simulink model "PMDC_exhibition"  (R2023b)
settings: Solver=VariableStepAuto  StartTime=0.0  StopTime=140  RelTol=1e-3
undefined symbols (not defined in the file or in its folder): B, dt, dT, J, Ke, Kt, L, LoadMode, R, Ro, SlopeR, Ts, Vp, Vs
libraries: simulink x1
settings Model: Creator=yanqi  LastModifiedBy=Brian Cheng

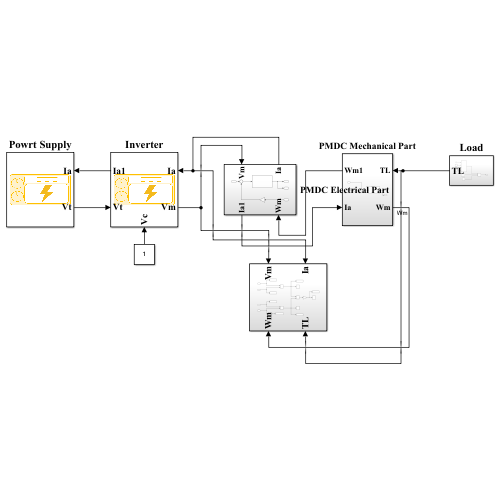
[thumbnail: Simulink's stored preview of the top-level diagram]
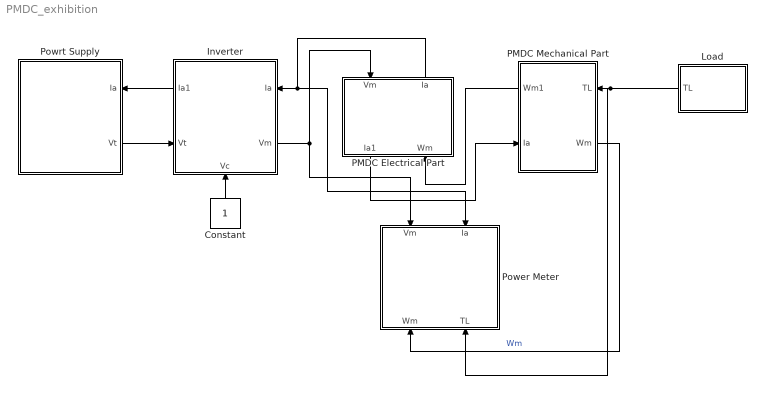
== system PMDC_exhibition ==
  Constant : Constant
  Inverter : Subsystem  InitFcn=Vp = 1;
      settings: PortSchema="{\"entries\":[{\"content\":{\"sides\":[{\"content\":{\"connectorIds\":[\"Out2\",\"In1\"]},\"type\":\"ConnectorPlacement.EquallySpacedRectSide\",\"uuid\":\"717e91a0-288b-4ba5-84da-f262c24688bc\"},{\"content\":{\"connectorIds\":[\"In3\",\"Out1\"],\"side\":\"RIGHT\"},\"type\":\"ConnectorPlacement.EquallySpacedRectSide\",\"uuid\":\"569ee505-38fb-400b-9e45-0fafedafb0f3\"},{\"content\":{\"side\":\"TOP\"},\"type\":\"ConnectorPlacement.EquallySpacedRectSide\",\"uuid\":\"44407c3d-239d-4fc9-b2d2-10ddbad2f525\"},{\"content\":{\"connectorIds\":[\"In2\"],\"side\":\"BOTTOM\"},\"type\":\"ConnectorPlacement.EquallySpacedRectSide\",\"uuid\":\"abc944a0-1837-407a-a5f0-1c34ab870232\"}]},\"type\":\"ConnectorPlacement.EquallySpacedConnector\",\"uuid\":\"e894aa65-7991-48d5-91da-50bab94327d3\"}],\"packageUris\":[\"http://schema.mathworks.com/mf0/Connector/R2020b\"],\"version\":\"1.0\"}"
      mask Display: image('$imagefile');
  Load : Subsystem  InitFcn=|
      | dt = 0.2;
      | dT = 0.05;
      | Ts = 2;
      | SlopeR = 0.2;
      | % if LoadMode>1.5, then use stair load
      | % if LoadMode<1.5, use linear load
      | LoadMode = 2;
  PMDC Electrical Part : Subsystem  InitFcn=|
      | % a=100
      | L = 0.0003137*a
      | R = 0.157378*a
      | J = 0.000466*a
      | B = 0.0002546*a
      | Ke = 0.0492*a
      | Kt = 0.0501*a
      settings: PortSchema="{\"entries\":[{\"content\":{\"sides\":[{\"content\":{\"connectorIds\":[\"Out2\",\"In1\"]},\"type\":\"ConnectorPlacement.EquallySpacedRectSide\",\"uuid\":\"0a5f02b8-770b-4e6c-8352-f728989d031b\"},{\"content\":{\"connectorIds\":[\"In2\",\"Out1\"],\"side\":\"RIGHT\"},\"type\":\"ConnectorPlacement.EquallySpacedRectSide\",\"uuid\":\"644f1108-5054-471c-8ace-4ff400685a6d\"},{\"content\":{\"connectorIds\":[],\"side\":\"TOP\"},\"type\":\"ConnectorPlacement.EquallySpacedRectSide\",\"uuid\":\"91f6ac77-69b1-43a4-9d17-8984b5c833f8\"}]},\"type\":\"ConnectorPlacement.EquallySpacedConnector\",\"uuid\":\"c8686663-a1fa-49f9-b914-1752eb8f4683\"}],\"packageUris\":[\"http://schema.mathworks.com/mf0/Connector/R2020b\"],\"version\":\"1.0\"}"
  PMDC Mechanical Part : Subsystem
      settings: PortSchema="{\"entries\":[{\"content\":{\"sides\":[{\"content\":{\"connectorIds\":[\"Out2\",\"In1\"]},\"type\":\"ConnectorPlacement.EquallySpacedRectSide\",\"uuid\":\"0a5f02b8-770b-4e6c-8352-f728989d031b\"},{\"content\":{\"connectorIds\":[\"In2\",\"Out1\"],\"side\":\"RIGHT\"},\"type\":\"ConnectorPlacement.EquallySpacedRectSide\",\"uuid\":\"644f1108-5054-471c-8ace-4ff400685a6d\"},{\"content\":{\"connectorIds\":[],\"side\":\"TOP\"},\"type\":\"ConnectorPlacement.EquallySpacedRectSide\",\"uuid\":\"91f6ac77-69b1-43a4-9d17-8984b5c833f8\"}]},\"type\":\"ConnectorPlacement.EquallySpacedConnector\",\"uuid\":\"c8686663-a1fa-49f9-b914-1752eb8f4683\"}],\"packageUris\":[\"http://schema.mathworks.com/mf0/Connector/R2020b\"],\"version\":\"1.0\"}"
  "Power Meter " : Subsystem  InitFcn=|  StopFcn=|
      InitFcn=|
      | %% ModePlot
      | % PlotMode=1 or 2
      | PlotMode = 2;
      StopFcn=|
      | % %% Data Loading
      | % 
      | % tl = out.Tl;
      | % f = size(tl);
      | % 
      | % % clear datas 
      | % torque = 0;
      | % y1 = 0; y2 = 0; y3 = 0; y4 = 0;
      | % 
      | % switch LoadMode   % mode ( 1:ramp load , 2:stair load )
      | % 
      | %     case 1  
      | % 
      | %         i = 1;
      | %         while 1
      | %             if tl(i) > 0.01
      | %                s = i;
      | %                break
      | %             end
      | %             i = i+1;
      | %         end
      | %         torque = out.Tl(s:f(1));
      | %         y1 = out.omega(s:f(1));
      | %         y2 = out.Eff(s:f(1));
      | %         y3 = out.Pin(s:f(1));
      | %         y4 = out.Pout(s:f(1));
      | %         case 2
      | % 
      | %         tl_pre = 0;
      | %         j = 1;
      | %         for i = 1:f(1)           
      | %             if tl(i) > tl_pre
      | %                 torque(j,1) = tl(i-1);
      | %                 y1(j,1) = out.omega((i-1),1);
      | %                 y2(j,1) = out.Eff((i-1),1);
      | %                 y3(j,1) = out.Pin((i-1),1);
      | %                 y4(j,1) = out.Pout((i-1),1);
      | %                 j = j+1;
      | %             end
      | %             tl_pre = tl(i);
      | %         end
      | % end
      | % 
      | % %% Plot
      | % % plot TN curve
      | % 
      | % figure(1);
      | % 
      | % % figure(2);
      | % clf;
      | % 
      | % % Create empty axis system with 4 y axis by calling:
      | % % handle = maxis(number of axis, y-spacing between outside lines)
      | % h = myaxisc(4,0.10,[0.1,0.1,0.8,0.8]); % Specify position
      | % 
      | % % Call plot and specify y-axis number using method h.p(nr). For creating a
      | % % legend later, we need to assign the handles returned by plot to p.
      | % switch PlotMode
      | % 
      | %     case 1  
      | %         p(1) = plot(h.p(1),torque,y1,'b','LineWidth',1.2);
      | %         p(2) = plot(h.p(2),torque,y2,'Color',[0.4660 0.6740 0.1880],'LineWidth',1.2);
      | %         p(3) = plot(h.p(3),torque,y3,'r','LineWidth',1.2);
      | %         p(4) = plot(h.p(4),torque,y4,'Color',[0.9290 0.6940 0.1250],'LineWidth',1.2);
      | %         print("case1");
      | % 
      | %     case 2
      | %         p(1) = plot(h.p(1),torque,y1,'b-*','LineWidth',1.1);
      | %         p(2) = plot(h.p(2),torque,y2,'-*','Color',[0.4660 0.6740 0.1880],'LineWidth',1.1);
      | %         p(3) = plot(h.p(3),torque,y3,'r-*','LineWidth',1.1);
      | %         p(4) = plot(h.p(4),torque,y4,'-*','Color',[0.9290 0.6940 0.1250],'LineWidth',1.1);
      | %         print("case2");
      | % 
      | % end
      | % 
      | % h.autoscale % Automatically Scale Y Axis
      | % 
      | % % Additional methods to modify appearance, scaling and so on:
      | % 
      | % h.autoy(3) % Autoscale only specified y-axis
      | % %h.ylim(3,[95,105]); % Set Y-Limits for axis 3
      | % l = size(torque);
      | % h.xlim([0,torque(l(1),1)+0.05]);
      | % h.ylim(2,[0,100]); % Set Y-Limits for axis 4
      | % 
      | % h.gridon % Enable grid (use h.gridoff to remove)
      | % 
      | % % Modify the y-Axis Color
      | % h.ycolor(1,'b');
      | % h.ycolor(2,[0.4660 0.6740 0.1880]);
      | % h.ycolor(3,'r');
      | % h.ycolor(4,[0.9290 0.6940 0.1250]);
      | % 
      | % % Add y-Labels
      | % h.ylabel(1,'Speed (RPM)');
      | % h.ylabel(2,'Efficiency (%)');
      | % h.ylabel(3,'Pin (W)');
      | % h.ylabel(4,'Pout (W)');
      | % 
      | % % Add x-Label
      | % h.xlabel('TL (Nm)');
      | % 
      | % % Change Position of the whole myaxisc-Object
      | % h.position([0.1,0.1,0.8,0.8],0.12); % Position-Vector and Spacing 0.12
      | % 
      | % % Change all font sizes
      | % h.fontsize(10)
      settings: PortSchema="{\"entries\":[{\"content\":{\"sides\":[{\"content\":{\"connectorIds\":[\"In1\",\"In2\"]},\"type\":\"ConnectorPlacement.EquallySpacedRectSide\",\"uuid\":\"e8c36156-32d4-4676-af0d-0891e0773ccb\"},{\"content\":{\"connectorIds\":[\"In3\",\"In4\"],\"side\":\"RIGHT\"},\"type\":\"ConnectorPlacement.EquallySpacedRectSide\",\"uuid\":\"5c876be3-b715-4990-b5f5-1fbda74411c9\"},{\"content\":{\"side\":\"TOP\"},\"type\":\"ConnectorPlacement.EquallySpacedRectSide\",\"uuid\":\"8aaa78a6-3767-49bf-860f-056d8a2101ef\"}]},\"type\":\"ConnectorPlacement.EquallySpacedConnector\",\"uuid\":\"6a38af7a-9eb4-49af-a88b-27cf70b05ead\"}],\"packageUris\":[\"http://schema.mathworks.com/mf0/Connector/R2020b\"],\"version\":\"1.0\"}"
  Powrt Supply : Subsystem  InitFcn=|
      | Vs = 110;
      | Ro = 0.001;
      settings: PortSchema="{\"entries\":[{\"content\":{\"sides\":[{\"content\":{},\"type\":\"ConnectorPlacement.EquallySpacedRectSide\",\"uuid\":\"717e91a0-288b-4ba5-84da-f262c24688bc\"},{\"content\":{\"connectorIds\":[\"In1\",\"Out1\"],\"side\":\"RIGHT\"},\"type\":\"ConnectorPlacement.EquallySpacedRectSide\",\"uuid\":\"569ee505-38fb-400b-9e45-0fafedafb0f3\"},{\"content\":{\"side\":\"TOP\"},\"type\":\"ConnectorPlacement.EquallySpacedRectSide\",\"uuid\":\"44407c3d-239d-4fc9-b2d2-10ddbad2f525\"}]},\"type\":\"ConnectorPlacement.EquallySpacedConnector\",\"uuid\":\"e894aa65-7991-48d5-91da-50bab94327d3\"}],\"packageUris\":[\"http://schema.mathworks.com/mf0/Connector/R2020b\"],\"version\":\"1.0\"}"
      mask Display: image('$imagefile');
  wires:
  Powrt Supply/1(Vt) -> Inverter/1(Vt)
  PMDC Electrical Part/2(Ia) -> "Power Meter "/1(Ia), Inverter/3(Ia)
  Inverter/1(Vm) -> "Power Meter "/2(Vm), PMDC Electrical Part/1(Vm)
  Load/1(TL) -> "Power Meter "/3(TL), PMDC Mechanical Part/2(TL)
  PMDC Mechanical Part/1(Wm) -> "Power Meter "/4(Wm)  "Wm"
  Constant/1 -> Inverter/2(Vc)
  Inverter/2(Ia1) -> Powrt Supply/1(Ia)
  PMDC Electrical Part/1(Ia1) -> PMDC Mechanical Part/1(Ia)
  PMDC Mechanical Part/2(Wm1) -> PMDC Electrical Part/2(Wm)

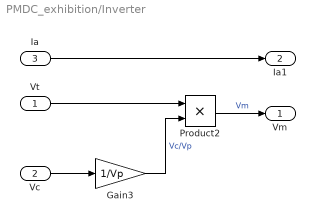
== system PMDC_exhibition/Inverter ==
  Vt : Inport
  Vc : Inport  Port=2
  Ia : Inport  Port=3
  Gain3 : Gain  Gain=1/Vp
  Product2 : Product
  Vm : Outport
  Ia1 : Outport  Port=2
  wires:
  Ia/1 -> Ia1/1
  Vc/1 -> Gain3/1
  Vt/1 -> Product2/1
  Product2/1 -> Vm/1  "Vm"
  Gain3/1 -> Product2/2  "Vc/Vp"

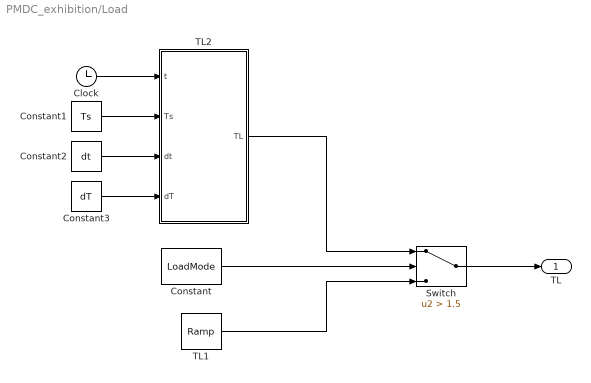
== system PMDC_exhibition/Load ==
  Clock : Clock
  Constant : Constant  Value=LoadMode
  Constant1 : Constant  Value=Ts
  Constant2 : Constant  Value=dt  SampleTime=dT
  Constant3 : Constant  Value=dT
  Switch : Switch  Criteria=u2 > Threshold  Threshold=1.5  SaturateOnIntegerOverflow=off  InputSameDT=off
  TL1 : simulink/Sources/Ramp  slope=SlopeR  start=Ts  InitialOutput=0
  TL2 : MATLAB Function  TreatAsAtomicUnit=on
  TL : Outport
  wires:
  Constant2/1 -> TL2/3(dt)
  Constant3/1 -> TL2/4(dT)
  Clock/1 -> TL2/1(t)
  Constant1/1 -> TL2/2(Ts)
  Switch/1 -> TL/1
  Constant/1 -> Switch/2
  TL2/1(TL) -> Switch/1
  TL1/1 -> Switch/3

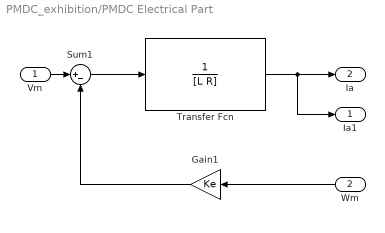
== system PMDC_exhibition/PMDC Electrical Part ==
  Vm : Inport
  Wm : Inport  Port=2
  Gain1 : Gain  Gain=Ke
  Sum1 : Sum  Inputs=|+-
  Transfer Fcn : TransferFcn  Denominator=[L R]
  Ia1 : Outport
  Ia : Outport  Port=2
  wires:
  Gain1/1 -> Sum1/2
  Sum1/1 -> Transfer Fcn/1
  Transfer Fcn/1 -> Ia1/1, Ia/1
  Wm/1 -> Gain1/1
  Vm/1 -> Sum1/1

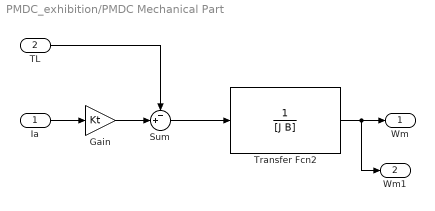
== system PMDC_exhibition/PMDC Mechanical Part ==
  Ia : Inport
  TL : Inport  Port=2
  Gain : Gain  Gain=Kt
  Sum : Sum  Inputs=-+|
  Transfer Fcn2 : TransferFcn  Denominator=[J B]
  Wm : Outport
  Wm1 : Outport  Port=2
  wires:
  Gain/1 -> Sum/2
  Ia/1 -> Gain/1
  Sum/1 -> Transfer Fcn2/1
  TL/1 -> Sum/1
  Transfer Fcn2/1 -> Wm1/1, Wm/1

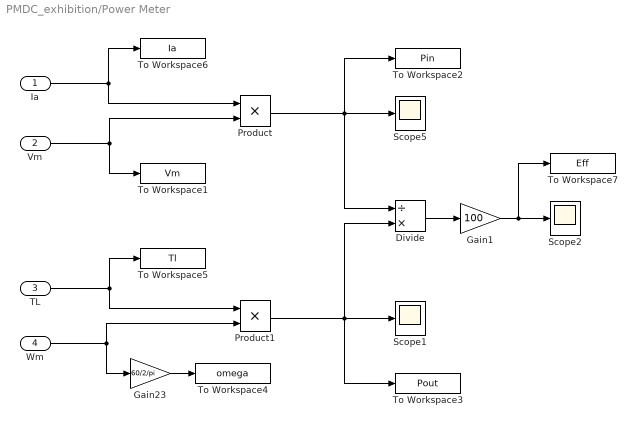
== system PMDC_exhibition/Power Meter  ==
  Ia : Inport
  Vm : Inport  Port=2
  TL : Inport  Port=3
  Wm : Inport  Port=4
  Divide : Product  Inputs=/*
  Gain1 : Gain  Gain=100
  Gain23 : Gain  Gain=60/2/pi
  Product : Product
  Product1 : Product
  Scope1 : Scope
  Scope2 : Scope
  Scope5 : Scope
  To Workspace1 : ToWorkspace  VariableName=Vm  SampleTime=-1
  To Workspace2 : ToWorkspace  VariableName=Pin  SampleTime=-1
  To Workspace3 : ToWorkspace  VariableName=Pout  SampleTime=-1
  To Workspace4 : ToWorkspace  VariableName=omega  SampleTime=-1
  To Workspace5 : ToWorkspace  VariableName=Tl  SampleTime=-1
  To Workspace6 : ToWorkspace  VariableName=Ia  SampleTime=-1
  To Workspace7 : ToWorkspace  VariableName=Eff  SampleTime=-1
  wires:
  Ia/1 -> Product/1, To Workspace6/1
  Vm/1 -> To Workspace1/1, Product/2
  Product/1 -> Divide/1, Scope5/1, To Workspace2/1
  Product1/1 -> Scope1/1, To Workspace3/1, Divide/2
  TL/1 -> To Workspace5/1, Product1/1
  Wm/1 -> Product1/2, Gain23/1
  Gain23/1 -> To Workspace4/1
  Divide/1 -> Gain1/1
  Gain1/1 -> To Workspace7/1, Scope2/1

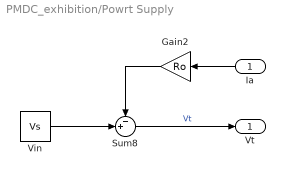
== system PMDC_exhibition/Powrt Supply ==
  Ia : Inport
  Gain2 : Gain  Gain=Ro
  Sum8 : Sum  Inputs=-+|
  Vin : Constant  Value=Vs
  Vt : Outport
  wires:
  Gain2/1 -> Sum8/1
  Sum8/1 -> Vt/1  "Vt"
  Vin/1 -> Sum8/2
  Ia/1 -> Gain2/1

== matlab function PMDC_exhibition/Load/TL2 ==
  data: t input; Ts input; TL output; dt input; dT input
function TL = fcn(t, Ts, dt, dT)

if t >= Ts
        TL = dT * fix((t-Ts)/dt);
else
    TL = 0;
end
